simulink model "ZweitankSystem_mit_regler"  (R2022a)
settings: Solver=VariableStepAuto  StartTime=0.0  StopTime=1000  RelTol=1e-3
values from neighbouring files (symbols this model uses):
  a = 1.963e-05    [Tank.m]
  G = 2*9.81    (= 19.62)    [Tank.m]
  iAt1 = 1/At1    (= 434.782608696)    [Tank.m]
  iAt2 = 1/At2    (= 256.41025641)    [Tank.m]
  K = 2.500e-06    (= 2.5e-06)    [Tank.m]
undefined symbols (not defined in the file or in its folder): sigbuilder_block
libraries: slpidlib x1
settings Model: Creator=Ibrahem  LastModifiedBy=Ibrahem

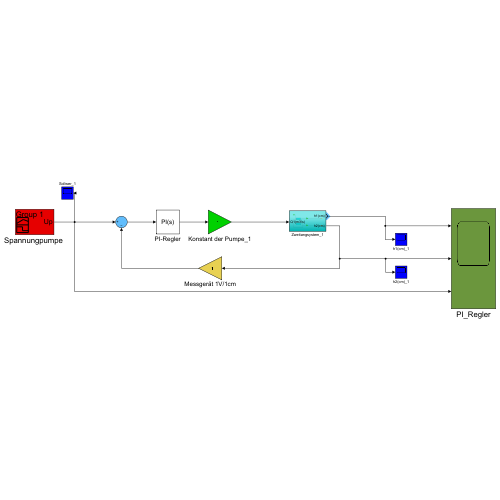
[thumbnail: Simulink's stored preview of the top-level diagram]
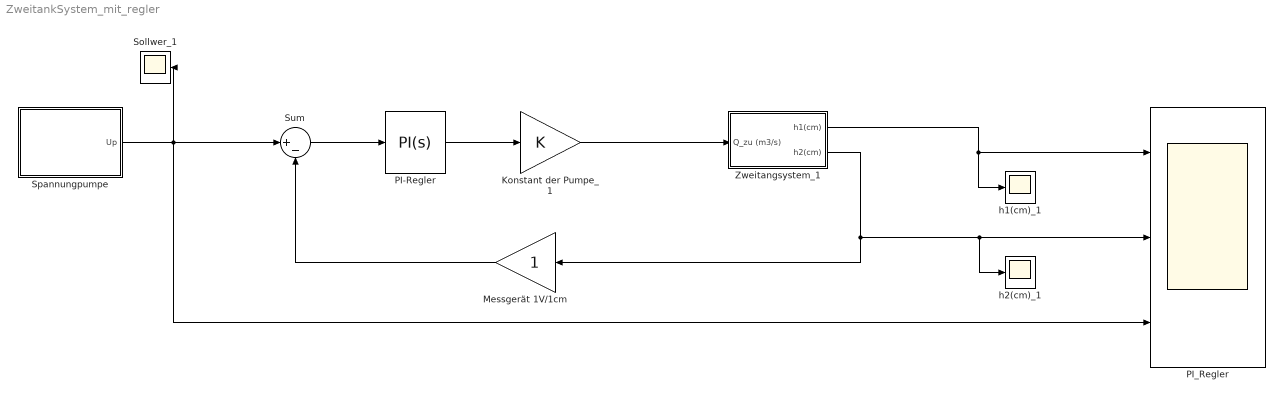
== system ZweitankSystem_mit_regler ==
  Konstant der Pumpe_1 : Gain  Gain=K
  Messgerät 1V/1cm : Gain
  PI-Regler : slpidlib/PID Controller  Controller=PI  Form=Ideal  TimeDomain=Continuous-time  UseExternalTs=off  SampleTime=-1  IntegratorMethod=Forward Euler  FilterMethod=Forward Euler  ControllerParametersSource=internal  P=7.25  I=1/25  UseKiTs=off  D=0  N=100  UseFilter=on  TunerSelectOption=Transfer Function Based (PID Tuner App)  InitialConditionSource=internal  InitialConditionForIntegrator=0  InitialConditionForFilter=0  DifferentiatorICPrevScaledInput=0  ExternalReset=none  TrackingMode=off  Kt=1  LimitOutput=off  SatLimitsSource=internal  UpperSaturationLimit=inf  LowerSaturationLimit=-inf  LinearizeAsGain=on  AntiWindupMode=none  Kb=1  POutMin=[]  POutMax=[]  IOutMin=[]  IOutMax=[]  DOutMin=[]  DOutMax=[]  NOutMin=[]  NOutMax=[]  SumOutMin=[]  SumOutMax=[]  SaturationOutMin=[]  SaturationOutMax=[]  PParamMin=[]  PParamMax=[]  IParamMin=[]  IParamMax=[]  DParamMin=[]  DParamMax=[]  NParamMin=[]  NParamMax=[]  KbParamMin=[]  KbParamMax=[]  KtParamMin=[]  KtParamMax=[]  KbOutMin=[]  KbOutMax=[]  KtOutMin=[]  KtOutMax=[]  IntegratorOutMin=[]  IntegratorOutMax=[]  FilterOutMin=[]  FilterOutMax=[]  SumI1OutMin=[]  SumI1OutMax=[]  SumI2OutMin=[]  SumI2OutMax=[]  SumI3OutMin=[]  SumI3OutMax=[]  SumI4OutMin=[]  SumI4OutMax=[]  SumDOutMin=[]  SumDOutMax=[]  DifferentiatorOutMin=[]  DifferentiatorOutMax=[]  FilterDiffOutCoefMin=[]  FilterDiffOutCoefMax=[]  ReciprocalOutMin=[]  ReciprocalOutMax=[]  SumDenOutMin=[]  SumDenOutMax=[]  SumNumOutMin=[]  SumNumOutMax=[]  DivideOutMin=[]  DivideOutMax=[]  UdiffTsProdOutMin=[]  UdiffTsProdOutMax=[]  NTsProdOutMin=[]  NTsProdOutMax=[]  UintegralTsProdOutMin=[]  UintegralTsProdOutMax=[]  UngainTsProdOutMin=[]  UngainTsProdOutMax=[]  IntegratorContinuousStateAttributes=''  IntegratorStateMustResolveToSignalObject=off  IntegratorRTWStateStorageClass=Auto  FilterContinuousStateAttributes=''  FilterStateMustResolveToSignalObject=off  FilterRTWStateStorageClass=Auto  ParallelPVariant=Passthrough  IdealPVariant=InternalParameters  IVariant=InternalParameters  DVariant=Disabled  IntegratorVariant=Continuous  SatVariant=Disabled  AWVariant=Passthrough  PCopyVariant=Disabled  TRVariant=Disabled  FdbkBlocksVariant=Forward  IdealPFdbkVariant=Disabled  SatFdbkVariant=Disabled  DerivativeFilterVariant=Disabled  NVariant=Disabled  NCopyVariant=Disabled_SignalSpec  FilterICVariant=Disabled  IntegratorICVariant=InternalICs  ExternalResetVariant=Disabled  TRSumVariant=Passthrough  SumFdbkVariant=Disabled  SumVariant=Sum_PI  TsampFilterVariant=InternalTs  TsampNgainVariant=Passthrough  TsampIntegralVariant=Passthrough  ExternalSaturationOutDataTypeStr=Inherit: Same as second input  aMode=0
  PI_Regler : Scope  NumInputPorts=3
  Sollwer_1 : Scope
  "Spannungpumpe " : Subsystem  Tag=STV Subsys  LoadFcn=sigbuilder_block('load');  StartFcn=sigbuilder_block('start');  StopFcn=sigbuilder_block('stop');  ClipboardFcn=sigbuilder_block('clipboard');  mask(Sigbuilder block){tuvar=[0:10]}
      mask help: Simulink:masks:SigbuilderBlock_MD
      mask init:
      | if ~strcmp(get_param(bdroot(gcbh),'SimulationStatus'),'stopped') tuvar = sigbuilder_block('maskInit'); end
      settings: CopyFcn=sigbuilder_block('copy');  DeleteFcn=sigbuilder_block('delete');  ModelCloseFcn=sigbuilder_block('modelClose');  PreSaveFcn=sigbuilder_block('preSave');  PauseFcn=sigbuilder_block('pause');  ContinueFcn=sigbuilder_block('continue');  NameChangeFcn=sigbuilder_block('namechange');  OpenFcn=sigbuilder_block('open',[5.5 30 949 418 ]);  CloseFcn=sigbuilder_block('close');
      mask Display: plot(0, 0, 100, 100,[2, 2, 32, 32, 2], [68, 8, 8, 68, 68],[32, 2], [38, 38], [32, 19, 2],[53, 60, 44], [32, 17, 17, 2],[16, 16, 31, 31]);txt = getActiveGroup(gcbh);text(2, 100, txt,'verticalAlignment', 'top');
  Sum : Sum  Inputs=|+-
  Zweitangsystem_1 : Subsystem
  h1(cm)_1 : Scope
  h2(cm)_1 : Scope
  wires:
  Zweitangsystem_1/2(h2(cm)) -> Messgerät 1V/1cm/1, PI_Regler/2, h2(cm)_1/1
  Messgerät 1V/1cm/1 -> Sum/2
  Konstant der Pumpe_1/1 -> Zweitangsystem_1/1(Q_zu (m3/s))
  Sum/1 -> PI-Regler/1
  PI-Regler/1 -> Konstant der Pumpe_1/1
  Zweitangsystem_1/1(h1(cm)) -> h1(cm)_1/1, PI_Regler/1
  "Spannungpumpe "/1(Up) -> Sollwer_1/1, Sum/1, PI_Regler/3

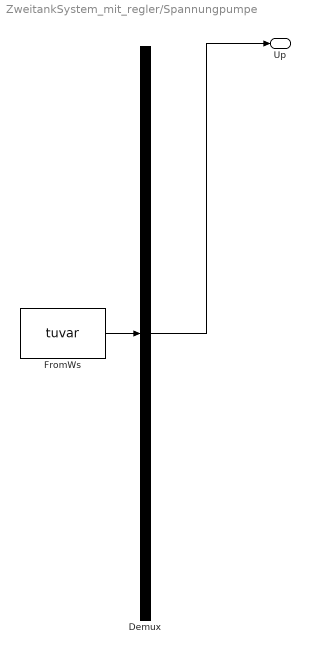
== system ZweitankSystem_mit_regler/Spannungpumpe  ==
  Demux : Demux  Tag=STV Demux  Outputs=1
      settings: DisplayOption=none
  FromWs : FromWorkspace  Tag=STV FromWs  VariableName=tuvar
      SigBuilderData=|
      | common.afterFinalStr = 'Extrapolate'
      | common.sampleTime = 0
      | dataSet.timeRange = [0 360]
      | dataSet.name = 'Group 1'
      | sbobj.Groups.Name = 'Group 1'
      | sbobj.Groups.Signals.Name = 'Up'
      | sbobj.Groups.Signals.XData = [0 100 100 300 300 360]
      | sbobj.Groups.Signals.YData = [1 0.98 4.98 4.98 2 2]
      | sbobj.Groups.TimeRange = [0 360]
  Up : Outport  Tag=STV Outport
  wires:
  FromWs/1 -> Demux/1
  Demux/1 -> Up/1

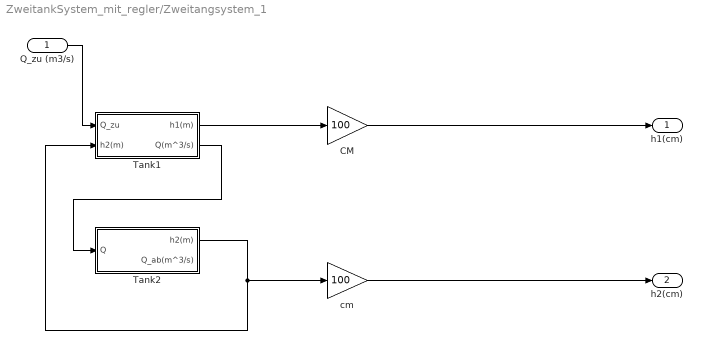
== system ZweitankSystem_mit_regler/Zweitangsystem_1 ==
  Q_zu (m3/s) : Inport
  CM : Gain  Gain=100
  Tank1 : Subsystem
  Tank2 : Subsystem
  cm : Gain  Gain=100
  h1(cm) : Outport
  h2(cm) : Outport  Port=2
  wires:
  Q_zu (m3/s)/1 -> Tank1/1(Q_zu)
  Tank2/1(h2(m)) -> Tank1/2(h2(m)), cm/1
  cm/1 -> h2(cm)/1
  Tank1/1(h1(m)) -> CM/1
  Tank1/2(Q(m^3/s)) -> Tank2/1(Q)
  CM/1 -> h1(cm)/1

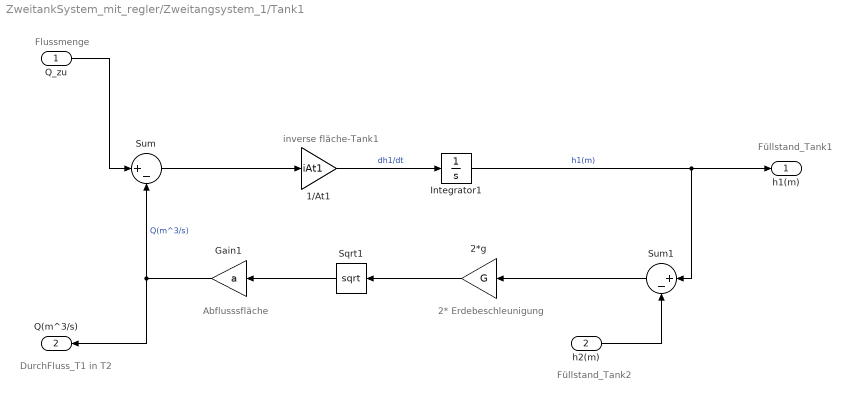
== system ZweitankSystem_mit_regler/Zweitangsystem_1/Tank1 ==
  note: inverse fläche-Tank1
  note: Abflusssfläche
  note: Flussmenge
  note: DurchFluss_T1 in T2
  note: 2* Erdebeschleunigung
  note: Füllstand_Tank1
  note: Füllstand_Tank2
  Q_zu : Inport
  h2(m) : Inport  Port=2
  1/At1 : Gain  Gain=iAt1
  2*g : Gain  Gain=G
  Gain1 : Gain  Gain=a
  Integrator1 : Integrator
  Sqrt1 : Sqrt
  Sum : Sum  Inputs=|+-
  Sum1 : Sum  Inputs=|+-
  h1(m) : Outport
  Q(m^3/s) : Outport  Port=2
  wires:
  2*g/1 -> Sqrt1/1
  h2(m)/1 -> Sum1/2
  1/At1/1 -> Integrator1/1  "dh1/dt"
  Gain1/1 -> Q(m^3/s)/1, Sum/2  "Q(m^3/s)"
  Integrator1/1 -> h1(m)/1, Sum1/1  "h1(m)"
  Sum/1 -> 1/At1/1
  Q_zu/1 -> Sum/1
  Sum1/1 -> 2*g/1
  Sqrt1/1 -> Gain1/1

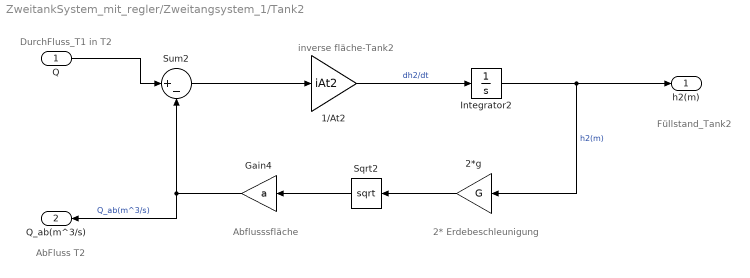
== system ZweitankSystem_mit_regler/Zweitangsystem_1/Tank2 ==
  note: DurchFluss_T1 in T2
  note: AbFluss T2
  note: inverse fläche-Tank2
  note: Abflusssfläche
  note: 2* Erdebeschleunigung
  note: Füllstand_Tank2
  Q : Inport
  1/At2 : Gain  Gain=iAt2
  2*g : Gain  Gain=G
  Gain4 : Gain  Gain=a
  Integrator2 : Integrator
  Sqrt2 : Sqrt
  Sum2 : Sum  Inputs=|+-
  h2(m) : Outport
  Q_ab(m^3/s) : Outport  Port=2
  wires:
  Sum2/1 -> 1/At2/1
  Integrator2/1 -> 2*g/1, h2(m)/1  "h2(m)"
  Sqrt2/1 -> Gain4/1
  Gain4/1 -> Q_ab(m^3/s)/1, Sum2/2  "Q_ab(m^3/s)"
  Q/1 -> Sum2/1
  1/At2/1 -> Integrator2/1  "dh2/dt"
  2*g/1 -> Sqrt2/1
